simulink library "VISMODAL_MASTER"  (Simulink 8.6)
settings: Solver=VariableStepAuto  StartTime=0.0  StopTime=10.0  RelTol=1e-3
libraries: VIS_LIB x140, cdsFilt x34, cdsMuxMatrix x6, VISMODAL_MASTER x1
(part 5 of 5)

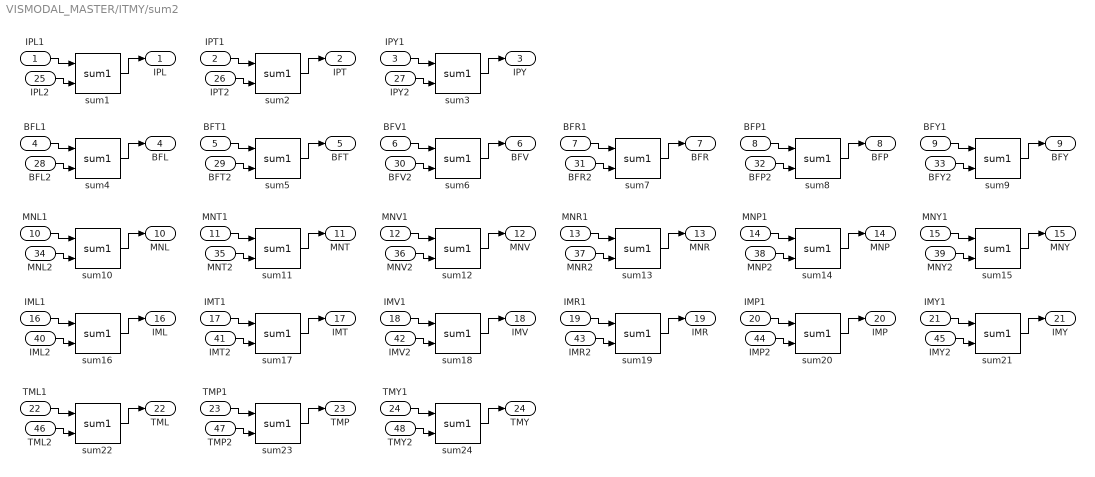
== system VISMODAL_MASTER/ITMY/sum2 ==
  IPL1 : Inport
  IPT1 : Inport  Port=2
  IPY1 : Inport  Port=3
  BFL1 : Inport  Port=4
  BFT1 : Inport  Port=5
  BFV1 : Inport  Port=6
  BFR1 : Inport  Port=7
  BFP1 : Inport  Port=8
  BFY1 : Inport  Port=9
  MNL1 : Inport  Port=10
  MNT1 : Inport  Port=11
  MNV1 : Inport  Port=12
  MNR1 : Inport  Port=13
  MNP1 : Inport  Port=14
  MNY1 : Inport  Port=15
  IML1 : Inport  Port=16
  IMT1 : Inport  Port=17
  IMV1 : Inport  Port=18
  IMR1 : Inport  Port=19
  IMP1 : Inport  Port=20
  IMY1 : Inport  Port=21
  TML1 : Inport  Port=22
  TMP1 : Inport  Port=23
  TMY1 : Inport  Port=24
  IPL2 : Inport  Port=25
  IPT2 : Inport  Port=26
  IPY2 : Inport  Port=27
  BFL2 : Inport  Port=28
  BFT2 : Inport  Port=29
  BFV2 : Inport  Port=30
  BFR2 : Inport  Port=31
  BFP2 : Inport  Port=32
  BFY2 : Inport  Port=33
  MNL2 : Inport  Port=34
  MNT2 : Inport  Port=35
  MNV2 : Inport  Port=36
  MNR2 : Inport  Port=37
  MNP2 : Inport  Port=38
  MNY2 : Inport  Port=39
  IML2 : Inport  Port=40
  IMT2 : Inport  Port=41
  IMV2 : Inport  Port=42
  IMR2 : Inport  Port=43
  IMP2 : Inport  Port=44
  IMY2 : Inport  Port=45
  TML2 : Inport  Port=46
  TMP2 : Inport  Port=47
  TMY2 : Inport  Port=48
  sum{1..24} (24 alike) : VIS_LIB/MODAL/sum1
  IPL : Outport
  IPT : Outport  Port=2
  IPY : Outport  Port=3
  BFL : Outport  Port=4
  BFT : Outport  Port=5
  BFV : Outport  Port=6
  BFR : Outport  Port=7
  BFP : Outport  Port=8
  BFY : Outport  Port=9
  MNL : Outport  Port=10
  MNT : Outport  Port=11
  MNV : Outport  Port=12
  MNR : Outport  Port=13
  MNP : Outport  Port=14
  MNY : Outport  Port=15
  IML : Outport  Port=16
  IMT : Outport  Port=17
  IMV : Outport  Port=18
  IMR : Outport  Port=19
  IMP : Outport  Port=20
  IMY : Outport  Port=21
  TML : Outport  Port=22
  TMP : Outport  Port=23
  TMY : Outport  Port=24
  wires:
  sum1/1 -> IPL/1
  IPL1/1 -> sum1/1
  sum2/1 -> IPT/1
  IPT1/1 -> sum2/1
  sum3/1 -> IPY/1
  IPY1/1 -> sum3/1
  sum4/1 -> BFL/1
  BFL1/1 -> sum4/1
  sum5/1 -> BFT/1
  BFT1/1 -> sum5/1
  sum6/1 -> BFV/1
  BFV1/1 -> sum6/1
  sum7/1 -> BFR/1
  BFR1/1 -> sum7/1
  sum8/1 -> BFP/1
  BFP1/1 -> sum8/1
  sum9/1 -> BFY/1
  BFY1/1 -> sum9/1
  sum10/1 -> MNL/1
  MNL1/1 -> sum10/1
  sum11/1 -> MNT/1
  MNT1/1 -> sum11/1
  sum12/1 -> MNV/1
  MNV1/1 -> sum12/1
  sum13/1 -> MNR/1
  MNR1/1 -> sum13/1
  sum14/1 -> MNP/1
  MNP1/1 -> sum14/1
  sum15/1 -> MNY/1
  MNY1/1 -> sum15/1
  sum16/1 -> IML/1
  IML1/1 -> sum16/1
  sum17/1 -> IMT/1
  IMT1/1 -> sum17/1
  sum18/1 -> IMV/1
  IMV1/1 -> sum18/1
  sum19/1 -> IMR/1
  IMR1/1 -> sum19/1
  sum20/1 -> IMP/1
  IMP1/1 -> sum20/1
  sum21/1 -> IMY/1
  IMY1/1 -> sum21/1
  sum22/1 -> TML/1
  TML1/1 -> sum22/1
  sum23/1 -> TMP/1
  TMP1/1 -> sum23/1
  sum24/1 -> TMY/1
  TMY1/1 -> sum24/1
  IPL2/1 -> sum1/2
  IPT2/1 -> sum2/2
  IPY2/1 -> sum3/2
  BFL2/1 -> sum4/2
  BFT2/1 -> sum5/2
  BFV2/1 -> sum6/2
  BFR2/1 -> sum7/2
  BFP2/1 -> sum8/2
  BFY2/1 -> sum9/2
  MNL2/1 -> sum10/2
  MNT2/1 -> sum11/2
  MNV2/1 -> sum12/2
  MNR2/1 -> sum13/2
  MNP2/1 -> sum14/2
  MNY2/1 -> sum15/2
  IML2/1 -> sum16/2
  IMT2/1 -> sum17/2
  IMV2/1 -> sum18/2
  IMR2/1 -> sum19/2
  IMP2/1 -> sum20/2
  IMY2/1 -> sum21/2
  TML2/1 -> sum22/2
  TMP2/1 -> sum23/2
  TMY2/1 -> sum24/2

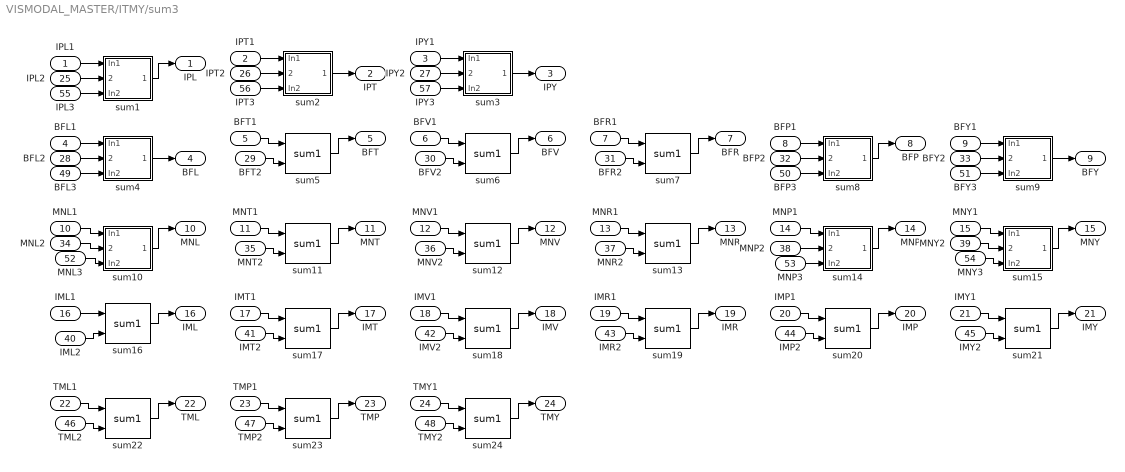
== system VISMODAL_MASTER/ITMY/sum3 ==
  IPL1 : Inport
  IPT1 : Inport  Port=2
  IPY1 : Inport  Port=3
  BFL1 : Inport  Port=4
  BFT1 : Inport  Port=5
  BFV1 : Inport  Port=6
  BFR1 : Inport  Port=7
  BFP1 : Inport  Port=8
  BFY1 : Inport  Port=9
  MNL1 : Inport  Port=10
  MNT1 : Inport  Port=11
  MNV1 : Inport  Port=12
  MNR1 : Inport  Port=13
  MNP1 : Inport  Port=14
  MNY1 : Inport  Port=15
  IML1 : Inport  Port=16
  IMT1 : Inport  Port=17
  IMV1 : Inport  Port=18
  IMR1 : Inport  Port=19
  IMP1 : Inport  Port=20
  IMY1 : Inport  Port=21
  TML1 : Inport  Port=22
  TMP1 : Inport  Port=23
  TMY1 : Inport  Port=24
  IPL2 : Inport  Port=25
  IPT2 : Inport  Port=26
  IPY2 : Inport  Port=27
  BFL2 : Inport  Port=28
  BFT2 : Inport  Port=29
  BFV2 : Inport  Port=30
  BFR2 : Inport  Port=31
  BFP2 : Inport  Port=32
  BFY2 : Inport  Port=33
  MNL2 : Inport  Port=34
  MNT2 : Inport  Port=35
  MNV2 : Inport  Port=36
  MNR2 : Inport  Port=37
  MNP2 : Inport  Port=38
  MNY2 : Inport  Port=39
  IML2 : Inport  Port=40
  IMT2 : Inport  Port=41
  IMV2 : Inport  Port=42
  IMR2 : Inport  Port=43
  IMP2 : Inport  Port=44
  IMY2 : Inport  Port=45
  TML2 : Inport  Port=46
  TMP2 : Inport  Port=47
  TMY2 : Inport  Port=48
  BFL3 : Inport  Port=49
  BFP3 : Inport  Port=50
  BFY3 : Inport  Port=51
  MNL3 : Inport  Port=52
  MNP3 : Inport  Port=53
  MNY3 : Inport  Port=54
  IPL3 : Inport  Port=55
  IPT3 : Inport  Port=56
  IPY3 : Inport  Port=57
  sum1 : Subsystem
  sum10 : Subsystem
  sum{5..7,11..13,16..24} (15 alike) : VIS_LIB/MODAL/sum1
  sum14 : Subsystem
  sum15 : Subsystem
  sum2 : Subsystem
  sum3 : Subsystem
  sum4 : Subsystem
  sum8 : Subsystem
  sum9 : Subsystem
  IPL : Outport
  IPT : Outport  Port=2
  IPY : Outport  Port=3
  BFL : Outport  Port=4
  BFT : Outport  Port=5
  BFV : Outport  Port=6
  BFR : Outport  Port=7
  BFP : Outport  Port=8
  BFY : Outport  Port=9
  MNL : Outport  Port=10
  MNT : Outport  Port=11
  MNV : Outport  Port=12
  MNR : Outport  Port=13
  MNP : Outport  Port=14
  MNY : Outport  Port=15
  IML : Outport  Port=16
  IMT : Outport  Port=17
  IMV : Outport  Port=18
  IMR : Outport  Port=19
  IMP : Outport  Port=20
  IMY : Outport  Port=21
  TML : Outport  Port=22
  TMP : Outport  Port=23
  TMY : Outport  Port=24
  wires:
  sum1/1(Out1) -> IPL/1
  IPL1/1 -> sum1/1(In1)
  sum2/1(Out1) -> IPT/1
  IPT1/1 -> sum2/1(In1)
  BFL1/1 -> sum4/1(In1)
  sum5/1 -> BFT/1
  BFT1/1 -> sum5/1
  sum6/1 -> BFV/1
  BFV1/1 -> sum6/1
  sum7/1 -> BFR/1
  BFR1/1 -> sum7/1
  sum8/1(Out1) -> BFP/1
  BFP1/1 -> sum8/1(In1)
  sum9/1(Out1) -> BFY/1
  BFY1/1 -> sum9/1(In1)
  sum10/1(Out1) -> MNL/1
  MNL1/1 -> sum10/1(In1)
  sum11/1 -> MNT/1
  MNT1/1 -> sum11/1
  sum12/1 -> MNV/1
  MNV1/1 -> sum12/1
  sum13/1 -> MNR/1
  MNR1/1 -> sum13/1
  sum14/1(Out1) -> MNP/1
  MNP1/1 -> sum14/1(In1)
  sum15/1(Out1) -> MNY/1
  MNY1/1 -> sum15/1(In1)
  sum16/1 -> IML/1
  IML1/1 -> sum16/1
  sum17/1 -> IMT/1
  IMT1/1 -> sum17/1
  sum18/1 -> IMV/1
  IMV1/1 -> sum18/1
  sum19/1 -> IMR/1
  IMR1/1 -> sum19/1
  sum20/1 -> IMP/1
  IMP1/1 -> sum20/1
  sum21/1 -> IMY/1
  IMY1/1 -> sum21/1
  sum22/1 -> TML/1
  TML1/1 -> sum22/1
  sum23/1 -> TMP/1
  TMP1/1 -> sum23/1
  sum24/1 -> TMY/1
  TMY1/1 -> sum24/1
  IPL2/1 -> sum1/2(In12)
  IPT2/1 -> sum2/2(In12)
  BFT2/1 -> sum5/2
  BFV2/1 -> sum6/2
  BFR2/1 -> sum7/2
  BFY2/1 -> sum9/2(In12)
  MNL2/1 -> sum10/2(In12)
  MNT2/1 -> sum11/2
  MNV2/1 -> sum12/2
  MNR2/1 -> sum13/2
  MNY2/1 -> sum15/2(In12)
  IML2/1 -> sum16/2
  IMT2/1 -> sum17/2
  IMV2/1 -> sum18/2
  IMR2/1 -> sum19/2
  IMP2/1 -> sum20/2
  IMY2/1 -> sum21/2
  TML2/1 -> sum22/2
  TMP2/1 -> sum23/2
  TMY2/1 -> sum24/2
  sum4/1(Out1) -> BFL/1
  BFL2/1 -> sum4/2(In12)
  BFP2/1 -> sum8/2(In12)
  MNP2/1 -> sum14/2(In12)
  BFY3/1 -> sum9/3(In2)
  BFL3/1 -> sum4/3(In2)
  BFP3/1 -> sum8/3(In2)
  MNL3/1 -> sum10/3(In2)
  MNY3/1 -> sum15/3(In2)
  MNP3/1 -> sum14/3(In2)
  IPY1/1 -> sum3/1(In1)
  IPY2/1 -> sum3/2(In12)
  sum3/1(Out1) -> IPY/1
  IPL3/1 -> sum1/3(In2)
  IPT3/1 -> sum2/3(In2)
  IPY3/1 -> sum3/3(In2)

== system VISMODAL_MASTER/ITMY/GASDC/SETPOINT ==
  LEN_IN : Inport
  TRA_IN : Inport  Port=2
  VER_IN : Inport  Port=3
  ROL_IN : Inport  Port=4
  PIT_IN : Inport  Port=5
  BF : cdsFilt/Subsystem  Tag=cdsFilt  Description=|
      | Purpose:                                                                                                                                                                                                                                  
      | Standard CDS IIR filter module.                                                                                                                                                                                                           
      |                                                                                                                                                                                                                                           
      | Operation:                                                                                                                                                                                                                                
      | Consists of 10 second order section IIR filters, plus a ramped gain stage. In FE code, also provides pre-defined test points and excitation channel inputs. The filter coefficients are defined in the LIGO system using the 'foton' tool.
      |                                                                                                                                                                                                                                           
      | Usage:                                                                                                                                                                                                                                    
      | Name the part with the desired filter module name.
      settings: AttributesFormatString=%<Tag>
  F0 : cdsFilt/Subsystem  Tag=cdsFilt  Description=|
      | Purpose:                                                                                                                                                                                                                                  
      | Standard CDS IIR filter module.                                                                                                                                                                                                           
      |                                                                                                                                                                                                                                           
      | Operation:                                                                                                                                                                                                                                
      | Consists of 10 second order section IIR filters, plus a ramped gain stage. In FE code, also provides pre-defined test points and excitation channel inputs. The filter coefficients are defined in the LIGO system using the 'foton' tool.
      |                                                                                                                                                                                                                                           
      | Usage:                                                                                                                                                                                                                                    
      | Name the part with the desired filter module name.
      settings: AttributesFormatString=%<Tag>
  F1 : cdsFilt/Subsystem  Tag=cdsFilt  Description=|
      | Purpose:                                                                                                                                                                                                                                  
      | Standard CDS IIR filter module.                                                                                                                                                                                                           
      |                                                                                                                                                                                                                                           
      | Operation:                                                                                                                                                                                                                                
      | Consists of 10 second order section IIR filters, plus a ramped gain stage. In FE code, also provides pre-defined test points and excitation channel inputs. The filter coefficients are defined in the LIGO system using the 'foton' tool.
      |                                                                                                                                                                                                                                           
      | Usage:                                                                                                                                                                                                                                    
      | Name the part with the desired filter module name.
      settings: AttributesFormatString=%<Tag>
  F2 : cdsFilt/Subsystem  Tag=cdsFilt  Description=|
      | Purpose:                                                                                                                                                                                                                                  
      | Standard CDS IIR filter module.                                                                                                                                                                                                           
      |                                                                                                                                                                                                                                           
      | Operation:                                                                                                                                                                                                                                
      | Consists of 10 second order section IIR filters, plus a ramped gain stage. In FE code, also provides pre-defined test points and excitation channel inputs. The filter coefficients are defined in the LIGO system using the 'foton' tool.
      |                                                                                                                                                                                                                                           
      | Usage:                                                                                                                                                                                                                                    
      | Name the part with the desired filter module name.
      settings: AttributesFormatString=%<Tag>
  F3 : cdsFilt/Subsystem  Tag=cdsFilt  Description=|
      | Purpose:                                                                                                                                                                                                                                  
      | Standard CDS IIR filter module.                                                                                                                                                                                                           
      |                                                                                                                                                                                                                                           
      | Operation:                                                                                                                                                                                                                                
      | Consists of 10 second order section IIR filters, plus a ramped gain stage. In FE code, also provides pre-defined test points and excitation channel inputs. The filter coefficients are defined in the LIGO system using the 'foton' tool.
      |                                                                                                                                                                                                                                           
      | Usage:                                                                                                                                                                                                                                    
      | Name the part with the desired filter module name.
      settings: AttributesFormatString=%<Tag>
  LEN_OUT : Outport
  TRA_OUT : Outport  Port=2
  VER_OUT : Outport  Port=3
  ROL_OUT : Outport  Port=4
  PIT_OUT : Outport  Port=5
  wires:
  F2/1 -> VER_OUT/1
  VER_IN/1 -> F2/1
  TRA_IN/1 -> F1/1
  F1/1 -> TRA_OUT/1
  F3/1 -> ROL_OUT/1
  ROL_IN/1 -> F3/1
  PIT_IN/1 -> BF/1
  BF/1 -> PIT_OUT/1
  LEN_IN/1 -> F0/1
  F0/1 -> LEN_OUT/1

== system VISMODAL_MASTER/ITMY/IPDC/SETPOINT ==
  LEN_IN : Inport
  PIT_IN : Inport  Port=2
  YAW_IN : Inport  Port=3
  LEN : cdsFilt/Subsystem  Tag=cdsFilt  Description=|
      | Purpose:                                                                                                                                                                                                                                  
      | Standard CDS IIR filter module.                                                                                                                                                                                                           
      |                                                                                                                                                                                                                                           
      | Operation:                                                                                                                                                                                                                                
      | Consists of 10 second order section IIR filters, plus a ramped gain stage. In FE code, also provides pre-defined test points and excitation channel inputs. The filter coefficients are defined in the LIGO system using the 'foton' tool.
      |                                                                                                                                                                                                                                           
      | Usage:                                                                                                                                                                                                                                    
      | Name the part with the desired filter module name.
      settings: AttributesFormatString=%<Tag>
  TRA : cdsFilt/Subsystem  Tag=cdsFilt  Description=|
      | Purpose:                                                                                                                                                                                                                                  
      | Standard CDS IIR filter module.                                                                                                                                                                                                           
      |                                                                                                                                                                                                                                           
      | Operation:                                                                                                                                                                                                                                
      | Consists of 10 second order section IIR filters, plus a ramped gain stage. In FE code, also provides pre-defined test points and excitation channel inputs. The filter coefficients are defined in the LIGO system using the 'foton' tool.
      |                                                                                                                                                                                                                                           
      | Usage:                                                                                                                                                                                                                                    
      | Name the part with the desired filter module name.
      settings: AttributesFormatString=%<Tag>
  YAW : cdsFilt/Subsystem  Tag=cdsFilt  Description=|
      | Purpose:                                                                                                                                                                                                                                  
      | Standard CDS IIR filter module.                                                                                                                                                                                                           
      |                                                                                                                                                                                                                                           
      | Operation:                                                                                                                                                                                                                                
      | Consists of 10 second order section IIR filters, plus a ramped gain stage. In FE code, also provides pre-defined test points and excitation channel inputs. The filter coefficients are defined in the LIGO system using the 'foton' tool.
      |                                                                                                                                                                                                                                           
      | Usage:                                                                                                                                                                                                                                    
      | Name the part with the desired filter module name.
      settings: AttributesFormatString=%<Tag>
  LEN_OUT : Outport
  PIT_OUT : Outport  Port=2
  YAW_OUT : Outport  Port=3
  wires:
  TRA/1 -> PIT_OUT/1
  PIT_IN/1 -> TRA/1
  YAW_IN/1 -> YAW/1
  YAW/1 -> YAW_OUT/1
  LEN_IN/1 -> LEN/1
  LEN/1 -> LEN_OUT/1

== system VISMODAL_MASTER/ITMY/TMOL/DC ==
  OLP : Inport
  OLY : Inport  Port=2
  BF : VIS_LIB/UTILs/FBs_2DOF
  Ground1 : Ground
  Ground3 : Ground
  MN : VIS_LIB/UTILs/FBs_2DOF
  SETPOINT : VIS_LIB/UTILs/FBs_2DOF
  Sum1 : Sum  Inputs=+-
  Sum2 : Sum  Inputs=+-
  BFP : Outport
  BFY : Outport  Port=2
  MNP : Outport  Port=3
  MNY : Outport  Port=4
  wires:
  OLP/1 -> Sum1/1
  Sum1/1 -> MN/1
  SETPOINT/1 -> Sum1/2
  OLY/1 -> Sum2/1
  Sum2/1 -> MN/2
  SETPOINT/2 -> Sum2/2
  Ground1/1 -> SETPOINT/1
  Ground3/1 -> SETPOINT/2
  BF/1 -> BFP/1
  BF/2 -> BFY/1
  MN/1 -> MNP/1, BF/1
  MN/2 -> MNY/1, BF/2

== system VISMODAL_MASTER/ITMY/TMOL/SERVO ==
  OLL : Inport
  OLP : Inport  Port=2
  OLY : Inport  Port=3
  BF : VIS_LIB/UTILs/FBs_3DOF_DQ
  IM : VIS_LIB/UTILs/FBs_3DOF_DQ
  MN : VIS_LIB/UTILs/FBs_3DOF_DQ
  TM : VIS_LIB/UTILs/FBs_3DOF_DQ
  BFL : Outport
  BFP : Outport  Port=2
  BFY : Outport  Port=3
  MNL : Outport  Port=4
  MNP : Outport  Port=5
  MNY : Outport  Port=6
  IML : Outport  Port=7
  IMP : Outport  Port=8
  IMY : Outport  Port=9
  TML : Outport  Port=10
  TMP : Outport  Port=11
  TMY : Outport  Port=12
  wires:
  OLL/1 -> BF/1, MN/1, IM/1, TM/1
  OLP/1 -> BF/2, MN/2, IM/2, TM/2
  OLY/1 -> BF/3, MN/3, IM/3, TM/3
  MN/1 -> MNL/1
  MN/2 -> MNP/1
  MN/3 -> MNY/1
  IM/1 -> IML/1
  IM/2 -> IMP/1
  IM/3 -> IMY/1
  TM/1 -> TML/1
  TM/2 -> TMP/1
  TM/3 -> TMY/1
  BF/1 -> BFL/1
  BF/2 -> BFP/1
  BF/3 -> BFY/1

== system VISMODAL_MASTER/ITMY/sum10/sum1 ==
  In1 : Inport
  In12 : Inport  Port=2
  In2 : Inport  Port=3
  Sum : Sum  Inputs=+++
  Out1 : Outport
  wires:
  In1/1 -> Sum/2
  In12/1 -> Sum/1
  Sum/1 -> Out1/1
  In2/1 -> Sum/3

== system VISMODAL_MASTER/ITMY/sum10/sum10 ==
  In1 : Inport
  In12 : Inport  Port=2
  In2 : Inport  Port=3
  Sum : Sum  Inputs=+++
  Out1 : Outport
  wires:
  In1/1 -> Sum/2
  In12/1 -> Sum/1
  Sum/1 -> Out1/1
  In2/1 -> Sum/3

== system VISMODAL_MASTER/ITMY/sum10/sum14 ==
  In1 : Inport
  In12 : Inport  Port=2
  In2 : Inport  Port=3
  Sum : Sum  Inputs=+++
  Out1 : Outport
  wires:
  In1/1 -> Sum/2
  In12/1 -> Sum/1
  Sum/1 -> Out1/1
  In2/1 -> Sum/3

== system VISMODAL_MASTER/ITMY/sum10/sum15 ==
  In1 : Inport
  In12 : Inport  Port=2
  In2 : Inport  Port=3
  Sum : Sum  Inputs=+++
  Out1 : Outport
  wires:
  In1/1 -> Sum/2
  In12/1 -> Sum/1
  Sum/1 -> Out1/1
  In2/1 -> Sum/3

== system VISMODAL_MASTER/ITMY/sum10/sum16 ==
  In1 : Inport
  In12 : Inport  Port=2
  In2 : Inport  Port=3
  Sum : Sum  Inputs=+++
  Out1 : Outport
  wires:
  In1/1 -> Sum/2
  In12/1 -> Sum/1
  Sum/1 -> Out1/1
  In2/1 -> Sum/3

== system VISMODAL_MASTER/ITMY/sum10/sum2 ==
  In1 : Inport
  In12 : Inport  Port=2
  In2 : Inport  Port=3
  Sum : Sum  Inputs=+++
  Out1 : Outport
  wires:
  In1/1 -> Sum/2
  In12/1 -> Sum/1
  Sum/1 -> Out1/1
  In2/1 -> Sum/3

== system VISMODAL_MASTER/ITMY/sum10/sum20 ==
  In1 : Inport
  In12 : Inport  Port=2
  In2 : Inport  Port=3
  Sum : Sum  Inputs=+++
  Out1 : Outport
  wires:
  In1/1 -> Sum/2
  In12/1 -> Sum/1
  Sum/1 -> Out1/1
  In2/1 -> Sum/3

== system VISMODAL_MASTER/ITMY/sum10/sum21 ==
  In1 : Inport
  In12 : Inport  Port=2
  In2 : Inport  Port=3
  Sum : Sum  Inputs=+++
  Out1 : Outport
  wires:
  In1/1 -> Sum/2
  In12/1 -> Sum/1
  Sum/1 -> Out1/1
  In2/1 -> Sum/3

== system VISMODAL_MASTER/ITMY/sum10/sum22 ==
  In1 : Inport
  In12 : Inport  Port=2
  In2 : Inport  Port=3
  Sum : Sum  Inputs=+++
  Out1 : Outport
  wires:
  In1/1 -> Sum/2
  In12/1 -> Sum/1
  Sum/1 -> Out1/1
  In2/1 -> Sum/3

== system VISMODAL_MASTER/ITMY/sum10/sum23 ==
  In1 : Inport
  In12 : Inport  Port=2
  In2 : Inport  Port=3
  Sum : Sum  Inputs=+++
  Out1 : Outport
  wires:
  In1/1 -> Sum/2
  In12/1 -> Sum/1
  Sum/1 -> Out1/1
  In2/1 -> Sum/3

== system VISMODAL_MASTER/ITMY/sum10/sum24 ==
  In1 : Inport
  In12 : Inport  Port=2
  In2 : Inport  Port=3
  Sum : Sum  Inputs=+++
  Out1 : Outport
  wires:
  In1/1 -> Sum/2
  In12/1 -> Sum/1
  Sum/1 -> Out1/1
  In2/1 -> Sum/3

== system VISMODAL_MASTER/ITMY/sum10/sum3 ==
  In1 : Inport
  In12 : Inport  Port=2
  In2 : Inport  Port=3
  Sum : Sum  Inputs=+++
  Out1 : Outport
  wires:
  In1/1 -> Sum/2
  In12/1 -> Sum/1
  Sum/1 -> Out1/1
  In2/1 -> Sum/3

== system VISMODAL_MASTER/ITMY/sum10/sum4 ==
  In1 : Inport
  In12 : Inport  Port=2
  In2 : Inport  Port=3
  Sum : Sum  Inputs=+++
  Out1 : Outport
  wires:
  In1/1 -> Sum/2
  In12/1 -> Sum/1
  Sum/1 -> Out1/1
  In2/1 -> Sum/3

== system VISMODAL_MASTER/ITMY/sum10/sum8 ==
  In1 : Inport
  In12 : Inport  Port=2
  In2 : Inport  Port=3
  Sum : Sum  Inputs=+++
  Out1 : Outport
  wires:
  In1/1 -> Sum/2
  In12/1 -> Sum/1
  Sum/1 -> Out1/1
  In2/1 -> Sum/3

== system VISMODAL_MASTER/ITMY/sum10/sum9 ==
  In1 : Inport
  In12 : Inport  Port=2
  In2 : Inport  Port=3
  Sum : Sum  Inputs=+++
  Out1 : Outport
  wires:
  In1/1 -> Sum/2
  In12/1 -> Sum/1
  Sum/1 -> Out1/1
  In2/1 -> Sum/3

== system VISMODAL_MASTER/ITMY/sum3/sum1 ==
  In1 : Inport
  In12 : Inport  Port=2
  In2 : Inport  Port=3
  Sum : Sum  Inputs=+++
  Out1 : Outport
  wires:
  In1/1 -> Sum/2
  In12/1 -> Sum/1
  Sum/1 -> Out1/1
  In2/1 -> Sum/3

== system VISMODAL_MASTER/ITMY/sum3/sum10 ==
  In1 : Inport
  In12 : Inport  Port=2
  In2 : Inport  Port=3
  Sum : Sum  Inputs=+++
  Out1 : Outport
  wires:
  In1/1 -> Sum/2
  In12/1 -> Sum/1
  Sum/1 -> Out1/1
  In2/1 -> Sum/3

== system VISMODAL_MASTER/ITMY/sum3/sum14 ==
  In1 : Inport
  In12 : Inport  Port=2
  In2 : Inport  Port=3
  Sum : Sum  Inputs=+++
  Out1 : Outport
  wires:
  In1/1 -> Sum/2
  In12/1 -> Sum/1
  Sum/1 -> Out1/1
  In2/1 -> Sum/3

== system VISMODAL_MASTER/ITMY/sum3/sum15 ==
  In1 : Inport
  In12 : Inport  Port=2
  In2 : Inport  Port=3
  Sum : Sum  Inputs=+++
  Out1 : Outport
  wires:
  In1/1 -> Sum/2
  In12/1 -> Sum/1
  Sum/1 -> Out1/1
  In2/1 -> Sum/3

== system VISMODAL_MASTER/ITMY/sum3/sum2 ==
  In1 : Inport
  In12 : Inport  Port=2
  In2 : Inport  Port=3
  Sum : Sum  Inputs=+++
  Out1 : Outport
  wires:
  In1/1 -> Sum/2
  In12/1 -> Sum/1
  Sum/1 -> Out1/1
  In2/1 -> Sum/3

== system VISMODAL_MASTER/ITMY/sum3/sum3 ==
  In1 : Inport
  In12 : Inport  Port=2
  In2 : Inport  Port=3
  Sum : Sum  Inputs=+++
  Out1 : Outport
  wires:
  In1/1 -> Sum/2
  In12/1 -> Sum/1
  Sum/1 -> Out1/1
  In2/1 -> Sum/3

== system VISMODAL_MASTER/ITMY/sum3/sum4 ==
  In1 : Inport
  In12 : Inport  Port=2
  In2 : Inport  Port=3
  Sum : Sum  Inputs=+++
  Out1 : Outport
  wires:
  In1/1 -> Sum/2
  In12/1 -> Sum/1
  Sum/1 -> Out1/1
  In2/1 -> Sum/3

== system VISMODAL_MASTER/ITMY/sum3/sum8 ==
  In1 : Inport
  In12 : Inport  Port=2
  In2 : Inport  Port=3
  Sum : Sum  Inputs=+++
  Out1 : Outport
  wires:
  In1/1 -> Sum/2
  In12/1 -> Sum/1
  Sum/1 -> Out1/1
  In2/1 -> Sum/3

== system VISMODAL_MASTER/ITMY/sum3/sum9 ==
  In1 : Inport
  In12 : Inport  Port=2
  In2 : Inport  Port=3
  Sum : Sum  Inputs=+++
  Out1 : Outport
  wires:
  In1/1 -> Sum/2
  In12/1 -> Sum/1
  Sum/1 -> Out1/1
  In2/1 -> Sum/3
